simulink model "VsourceInverter_Boost"  (R2017b)
settings: Solver=ode45  StartTime=0.0  StopTime=0.05  RelTol=1e-3  EnableMultiTasking=on
InitFcn:
  | FREQ = 85e3;
  | w = 2*pi*FREQ;
  | Vdc = 100;
  | Lp = 263e-6;
  | Ls =258e-6;
  | M = 60e-6;
  | Cp = 1/w^2/Lp;
  | Cs = 1/w^2/Ls;
libraries: powerlib x30, powerlib_meascontrol x8, simulink x3
settings Model: SimulationMode=accelerator  Creator=User  LastModifiedBy=SuperWindows
settings DataIOCC: FinalStateName=xInitial  LimitDataPoints=on  SaveFinalState=on  SaveFormat=Array
settings OptimizationCC: LifeSpan=inf
settings DebuggingCC: SolverPrmCheckMsg=warning  SFUnexpectedBacktrackingDiag=warning  SFNoUnconditionalDefaultTransitionDiag=warning  SFExecutionAtInitializationDiag=none
settings HardwareCC: ProdBitPerPointer=32  ProdBitPerSizeT=32  ProdBitPerPtrDiffT=32  ProdLargestAtomicFloat=None  ProdIntDivRoundTo=Undefined  ProdEndianess=Unspecified  ProdWordSize=32  ProdHWDeviceType=32-bit Generic
settings ModelReferenceCC: PropagateSignalLabelsOutOfModel=off
settings CodeAppCC: StateflowObjectComments=on
settings GRTTargetCC: TargetLangStandard=C89/C90 (ANSI)  GeneratePreprocessorConditionals=Disable all
settings ConfigComp: CovMetricSettings=dw  CovHtmlReporting=on  CovSaveCumulativeToWorkspaceVar=on  CovSaveSingleToWorkspaceVar=on  CovExternalEMLEnable=off  CovSFcnEnable=off
settings SimscapeCC: SimscapeNormalizeSystem=off

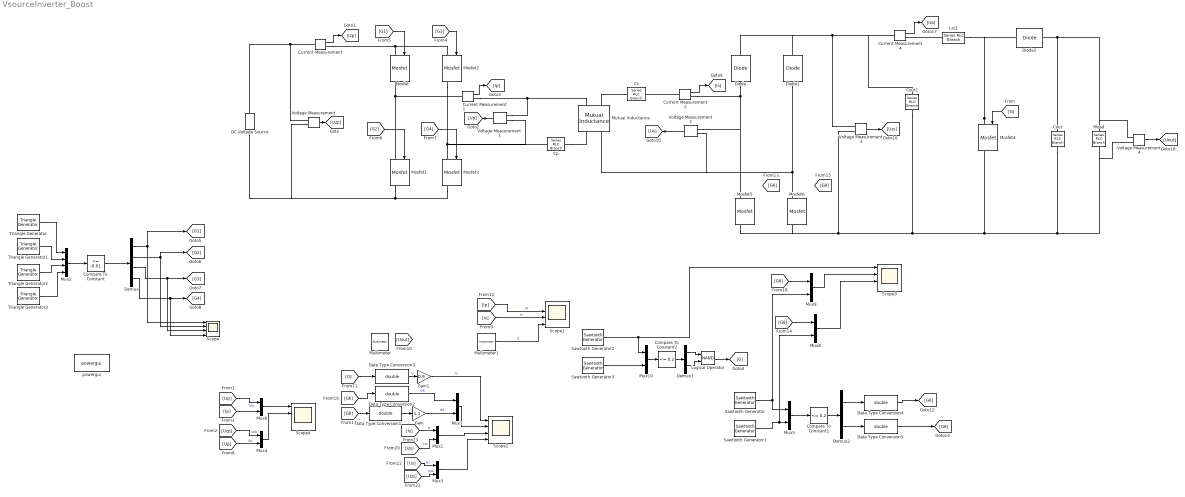
== system VsourceInverter_Boost ==
  Compare To Constant : simulink/Logic and Bit Operations/Compare To Constant  relop=<=  const=-0.01  OutDataTypeStr=boolean
  Compare To Constant1 : simulink/Logic and Bit Operations/Compare To Constant  relop=<=  const=0.2  OutDataTypeStr=uint8
  Compare To Constant2 : simulink/Logic and Bit Operations/Compare To Constant  relop=<=  const=0.2  OutDataTypeStr=uint8
  Cout : powerlib/Elements/Series RLC Branch  LConnTagsString=__new0  RConnTagsString=__new0  BranchType=C  Resistance=1  Inductance=1e-3  SetiL0=off  InitialCurrent=0  Capacitance=470e-6  Setx0=on  InitialVoltage=60  Measurements=Branch voltage and current
  Cout1 : powerlib/Elements/Series RLC Branch  LConnTagsString=__new0  RConnTagsString=__new0  BranchType=C  Resistance=1  Inductance=1e-3  SetiL0=off  InitialCurrent=0  Capacitance=470e-6  Setx0=on  InitialVoltage=60  Measurements=Branch voltage and current
  Cp : powerlib/Elements/Series RLC Branch  LConnTagsString=__new0  RConnTagsString=__new0  BranchType=RC  Resistance=0.02  Inductance=1e-3  SetiL0=off  InitialCurrent=0  Capacitance=Cp  Setx0=off  InitialVoltage=100  Measurements=Branch voltage and current
  Cs : powerlib/Elements/Series RLC Branch  LConnTagsString=__new0  RConnTagsString=__new0  BranchType=RC  Resistance=0.02  Inductance=1e-3  SetiL0=off  InitialCurrent=0  Capacitance=Cs  Setx0=off  InitialVoltage=100  Measurements=Branch voltage and current
  Current Measurement{,1,3..4} (4 alike) : powerlib/Measurements/Current Measurement  PhasorSimulation=off  OutputType=Complex  PSBequivalent=0
  DC Voltage Source : powerlib/Electrical Sources/DC Voltage Source  Amplitude=Vdc  Measurements=None
  Data Type Conversion{1..5} (5 alike) : DataTypeConversion  OutDataTypeStr=double
  Demux : Demux
  Demux1 : Demux  Outputs=2
  Demux2 : Demux  Outputs=2
  Diode : powerlib/Power Electronics/Diode  Ron=0.001  Lon=0  Vf=0.4  IC=0  UseSnubber=0  Rs=1e5  Cs=250e-9  Measurements=off
  Diode1 : powerlib/Power Electronics/Diode  Ron=0.001  Lon=0  Vf=0.4  IC=0  UseSnubber=0  Rs=1e5  Cs=250e-9  Measurements=off
  Diode2 : powerlib/Power Electronics/Diode  Ron=0.001  Lon=0  Vf=0.4  IC=0  UseSnubber=0  Rs=1e5  Cs=250e-9  Measurements=off
  Gain : Gain  Gain=1.1
  Gain1 : Gain  Gain=0.9
  Logical Operator : Logic  Operator=NAND  AllPortsSameDT=off  OutDataTypeStr=boolean
  Lsz1 : powerlib/Elements/Series RLC Branch  LConnTagsString=__new0  RConnTagsString=__new0  BranchType=L  Resistance=1  Inductance=3e-4  SetiL0=off  InitialCurrent=0  Capacitance=4700e-6  Setx0=on  InitialVoltage=60  Measurements=Branch voltage and current
  Mosfet{,1..6} (7 alike) : powerlib/Power Electronics/Mosfet  Ron=0.1  Lon=0  Rd=0.01  Vfd=0  IC=0  Rs=1e5  Cs=inf  Measurements=on
  Multimeter : powerlib/Measurements/Multimeter  PhasorSimulation=off  OutputType=Complex  sel=1  L=12  Gain=0  yselected={}  PSBOutputType=1  PSBequivalent=0  AxesSetting=[0,0.1,-100,100]  Display=0  SavedBlockNames=-11
  Multimeter1 : powerlib/Measurements/Multimeter  PhasorSimulation=off  OutputType=Complex  sel=1  L=12  Gain=0  yselected={}  PSBOutputType=1  PSBequivalent=0  AxesSetting=[0,0.1,-100,100]  Display=0  SavedBlockNames=-11
  Mutual Inductance : powerlib/Elements/Mutual Inductance  LConnTagsString=a|b  RConnTagsString=A|B  TypeOfMutual=Two or three windings with equal mutual terms  NumberOfWindings=3  SelfImpedance1=[0.22 Lp]  SelfImpedance2=[0.22 Ls]  ThreeWindings=off  SelfImpedance3=[ 1.1 1.1e-03]  MutualImpedance=[0 M]  InductanceMatrix="[1.0 0.9  0.9 ;  0.9 1.0  0.9;  0.9 0.9 1.0 ] * 1e-3"  ResistanceMatrix="[1.0 0.9  0.9 ;  0.9 1.0  0.9;  0.9 0.9 1.0 ]"  Measurements=None
      settings: AttributesFormatString=\n  SourceProductName=Simscape Power Systems  SourceProductBaseCode=PS
  Mux{1,3..10} (9 alike) : Mux  Inputs=2
  Mux2 : Mux
  Rload : powerlib/Elements/Series RLC Branch  LConnTagsString=__new0  RConnTagsString=__new0  BranchType=R  Resistance=40  Inductance=1e-3  SetiL0=off  InitialCurrent=0  Capacitance=470e-6  Setx0=off  InitialVoltage=100  Measurements=Branch voltage and current
  Sawtooth Generator : powerlib_meascontrol/Pulse & Signal Generators/Sawtooth Generator  Freq=FREQ  Phase=0  Ts=0
      settings: SourceProductName=Simscape Power Systems
  Sawtooth Generator1 : powerlib_meascontrol/Pulse & Signal Generators/Sawtooth Generator  Freq=FREQ  Phase=180  Ts=0
      settings: SourceProductName=Simscape Power Systems
  Sawtooth Generator2 : powerlib_meascontrol/Pulse & Signal Generators/Sawtooth Generator  Freq=FREQ  Phase=0  Ts=0
      settings: SourceProductName=Simscape Power Systems
  Sawtooth Generator3 : powerlib_meascontrol/Pulse & Signal Generators/Sawtooth Generator  Freq=FREQ  Phase=180  Ts=0
      settings: SourceProductName=Simscape Power Systems
  Scope{,1..4} (5 alike) : Scope  NumInputPorts=4
  Triangle Generator : powerlib_meascontrol/Pulse & Signal Generators/Triangle Generator  Freq=FREQ  Phase=0  Ts=0
  Triangle Generator1 : powerlib_meascontrol/Pulse & Signal Generators/Triangle Generator  Freq=FREQ  Phase=180  Ts=0
  Triangle Generator2 : powerlib_meascontrol/Pulse & Signal Generators/Triangle Generator  Freq=FREQ  Phase=180  Ts=0
  Triangle Generator3 : powerlib_meascontrol/Pulse & Signal Generators/Triangle Generator  Freq=FREQ  Phase=0  Ts=0
  Voltage Measurement{,1..4} (5 alike) : powerlib/Measurements/Voltage Measurement  PhasorSimulation=off  OutputType=Complex  PSBequivalent=0
  powergui : powerlib/powergui  Priority=1  SimulationMode=Discrete  SampleTime=1e-8  frequency=60  Iterations=50  frequencyindice=0  Pbase=100e6  ErrMax=1e-4  UnitsV=kV  UnitsW=MW  buscounter=0  FunctionMessages=off  echomessages=off  EnableUseOfTLC=off  CurrentSourceSwitches=off  DisableSnubberDevices=off  DisableRonSwitches=off  DisableVfSwitches=off  DisplayEquations=off  SolverType=Tustin/Backward Euler (TBE)  Interpol=off  ExternalGateDelay=off  methode=off  Ts=100  x0status=blocks  SPID=on  SwTol=0  HookPort=off  RestoreLinks=warning  ResistiveCurrentMeasurement=off  Frange=[0:2:500]  Ylog=off  Xlog=on  ShowGrid=off  save=off  variable=ZData  structure=0  ZoomFFT=off  StartTime=0.0  cycles=1  DisplayStyle=1  fundamental=60  FreqAxis=off  MaxFrequency=1000  frequencyindicesteady=1  RmsSteady=1  display=off
  wires:
  Voltage Measurement/1 -> [Uzp]
  Current Measurement/1 -> [Izp]
  Current Measurement1/1 -> [Ip]
  [G1] -> Mosfet/1
  [G4] -> Mosfet3/1
  [G2] -> Mosfet1/1
  [G3] -> Mosfet2/1
  Demux/1 -> [G1], Scope/1
  Demux/2 -> [G2], Scope/2
  Demux/3 -> Scope/3, [G3]
  Demux/4 -> Scope/4, [G4]
  Triangle Generator/1 -> Mux2/1
  Triangle Generator1/1 -> Mux2/2
  Triangle Generator2/1 -> Mux2/3
  Triangle Generator3/1 -> Mux2/4
  Mux2/1 -> Compare To Constant/1
  Compare To Constant/1 -> Demux/1
  Compare To Constant1/1 -> Demux2/1
  Mux5/1 -> Compare To Constant1/1
  Demux2/2 -> Data Type Conversion5/1
  Sawtooth Generator/1 -> Mux9/2, Mux5/1
  Sawtooth Generator1/1 -> Mux8/2, Mux5/2
  Voltage Measurement1/1 -> [Up]
  [Up] -> Mux4/2  "Up"
  Mux4/1 -> Scope4/2
  Current Measurement3/1 -> [Is]
  Voltage Measurement2/1 -> [Us]
  Voltage Measurement3/1 -> [Uzs]
  Current Measurement4/1 -> [Izs]
  Voltage Measurement4/1 -> [Uout]
  [Izs] -> Mux1/2  "Izs"
  [Is] -> Mux1/1  "Is"
  Mux1/1 -> Scope2/3
  [Us] -> Mux3/1  "Us"
  [Uzs] -> Mux3/2  "Uzs"
  Mux3/1 -> Scope2/4
  Mux6/1 -> Scope4/1
  [Izp] -> Mux6/1  "Idc"
  [Ip] -> Mux6/2
  [Uzp] -> Mux4/1  "Udc"
  [Is] -> Scope1/3  "Is"
  Multimeter1/1 -> Scope1/4  "IL"
  [G] -> Mosfet4/1
  [Ip] -> Scope1/2  "Ip"
  [G8] -> Data Type Conversion1/1
  Mux7/1 -> Scope2/2
  Data Type Conversion1/1 -> Gain/1
  Gain/1 -> Mux7/2  "G8"
  [G6] -> Data Type Conversion2/1
  Data Type Conversion2/1 -> Mux7/1  "G6"
  Demux2/1 -> Data Type Conversion4/1
  [G] -> Data Type Conversion3/1
  Data Type Conversion3/1 -> Gain1/1  "G"
  Gain1/1 -> Scope2/1  "G"
  Sawtooth Generator2/1 -> Mux10/1, Scope3/1
  [G8] -> Mux8/1
  [G6] -> Mux9/1
  Mux9/1 -> Scope3/2
  Mux8/1 -> Scope3/3
  Data Type Conversion4/1 -> [G6]
  Data Type Conversion5/1 -> [G8]
  Sawtooth Generator3/1 -> Mux10/2
  Mux10/1 -> Compare To Constant2/1
  Logical Operator/1 -> [G]
  Compare To Constant2/1 -> Demux1/1
  Demux1/2 -> Logical Operator/2
  Demux1/1 -> Logical Operator/1
  connections:
  Mosfet3/RConn1 -- Voltage Measurement/LConn2 -- DC Voltage Source/LConn1 -- Mosfet1/RConn1
  Current Measurement/LConn1 -- Voltage Measurement/LConn1 -- DC Voltage Source/RConn1
  Mosfet1/LConn1 -- Current Measurement1/LConn1 -- Mosfet/RConn1
  Mosfet2/RConn1 -- Cp/LConn1 -- Voltage Measurement1/LConn2 -- Mosfet3/LConn1
  Mosfet/LConn1 -- Mosfet2/LConn1 -- Current Measurement/RConn1
  Voltage Measurement1/LConn1 -- Current Measurement1/RConn1 -- Mutual Inductance/LConn1
  Cp/RConn1 -- Mutual Inductance/RConn1
  Cs/RConn1 -- Mutual Inductance/LConn2
  Mosfet5/LConn1 -- Voltage Measurement2/LConn1 -- Diode/LConn1 -- Current Measurement3/RConn1
  Mutual Inductance/RConn2 -- Voltage Measurement2/LConn2 -- Mosfet6/LConn1 -- Diode1/LConn1
  Mosfet6/RConn1 -- Mosfet5/RConn1 -- Cout1/RConn1 -- Mosfet4/RConn1 -- Voltage Measurement4/LConn2 -- Rload/RConn1 -- Cout/RConn1 -- Voltage Measurement3/LConn2
  Cout/LConn1 -- Voltage Measurement4/LConn1 -- Rload/LConn1 -- Diode2/RConn1
  Current Measurement3/LConn1 -- Cs/LConn1
  Diode1/RConn1 -- Diode/RConn1 -- Cout1/LConn1 -- Current Measurement4/LConn1 -- Voltage Measurement3/LConn1
  Mosfet4/LConn1 -- Lsz1/LConn1 -- Diode2/LConn1
  Lsz1/RConn1 -- Current Measurement4/RConn1
